simulink model "dvbs2_stream"  (R2024b)
settings: Solver=FixedStepDiscrete  StartTime=0.0  StopTime=18000/Fs  RelTol=1e-3
PreLoadFcn:
  | Rs = 125e3;
  | Fs = 8*Rs;
  | nsamp = 4096;
  | t = (0:nsamp)/Fs;
  | y = randi(2^8-1,1,2048);
  | ly = length(y);
InitFcn:
  | Rs = 125e3;
  | Fs = 8*Rs;
  | nsamp = 4096;
  | t = (0:nsamp)/Fs;
  | y = randi(2^8-1,1,2048);
  | ly = length(y);
libraries: hdlsllib x132, simulink x41, dspsigops x7, commseqgen3 x5, whdlutilities x5, commhdlcrc x2, dsphdlfiltering2 x1, whdlmod x1, sdrzblksprivate x1
(part 1 of 6)
CloseFcn:
  | clear Fs nsamp t y ly
settings Model: Creator=The MathWorks, Inc.  LastModifiedBy=daniel
settings SolverCC: AlgebraicLoopSolver=TrustRegion
settings OptimizationCC: BlockReduction=off  ConditionallyExecuteInputs=off  DefaultParameterBehavior=Inlined
settings DebuggingCC: AlgebraicLoopMsg=error  UnconnectedInputMsg=warning  UnconnectedOutputMsg=warning  UnconnectedLineMsg=warning
settings HardwareCC: ProdBitPerPointer=32  ProdBitPerSizeT=32  ProdBitPerPtrDiffT=32  ProdLargestAtomicFloat=None  ProdIntDivRoundTo=Undefined  ProdEndianess=Unspecified  ProdWordSize=32  ProdHWDeviceType=ASIC/FPGA->ASIC/FPGA  TargetBitPerLong=64  TargetBitPerPointer=64  TargetBitPerSizeT=64  TargetBitPerPtrDiffT=64  TargetLongLongMode=on  TargetIntDivRoundTo=Zero  TargetEndianess=LittleEndian  TargetWordSize=64  TargetHWDeviceType=Custom Processor->MATLAB Host Computer  ProdEqTarget=off
settings ModelReferenceCC: EnableRefExpFcnMdlSchedulingChecks=on
settings RTWCC: GPUComputeCapability=3.5

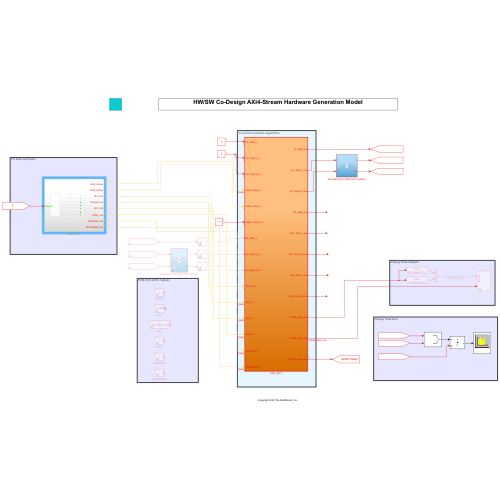
[thumbnail: Simulink's stored preview of the top-level diagram]
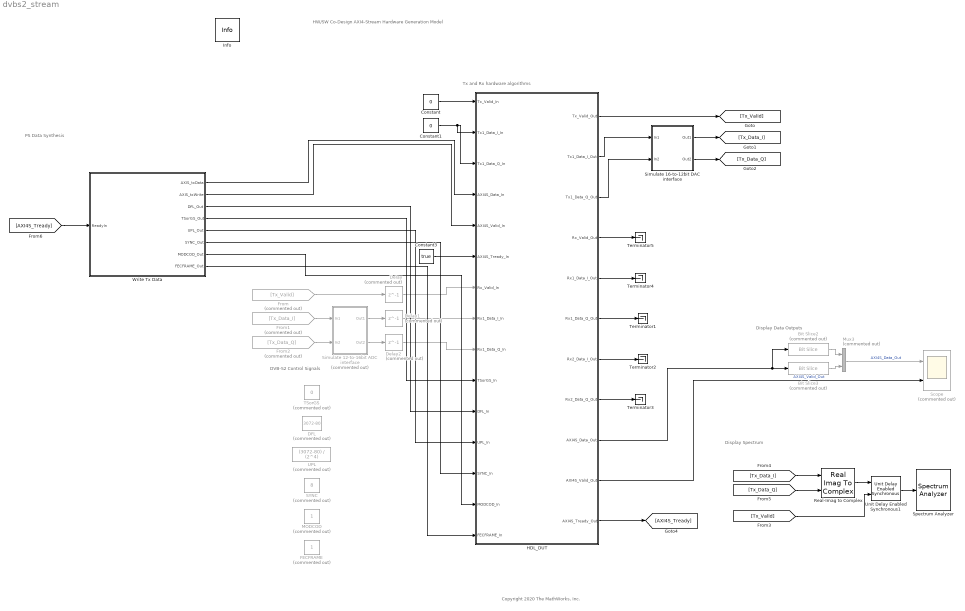
== system dvbs2_stream ==
  note: Tx and Rx hardware algorithms
  note: DVB-S2 Control Signals
  note: Display Data Outputs
  note: PS Data Synthesis
  note: HW/SW Co-Design AXI4-Stream Hardware Generation Model
  note: Copyright 2020 The MathWorks, Inc.
  note: Display Spectrum
  Bit Slice2 : hdlsllib/Logic and Bit Operations/Bit Slice  Commented=on  lidx=31  ridx=16
  Bit Slice3 : hdlsllib/Logic and Bit Operations/Bit Slice  Commented=on  lidx=15  ridx=0
  Constant : Constant  Value=0  OutDataTypeStr=boolean  SampleTime=-1
  Constant1 : Constant  Value=0  OutDataTypeStr=int16  SampleTime=-1
  Constant3 : Constant  Value=true  SampleTime=-1
  DFL : Constant  Commented=on  Value=3072-80  OutDataTypeStr=uint16  SampleTime=-1
  Delay : Delay  Commented=on  DelayLength=1
  Delay1 : Delay  Commented=on  DelayLength=1
  Delay2 : Delay  Commented=on  DelayLength=1
  FECFRAME : Constant  Commented=on  OutDataTypeStr=boolean  SampleTime=-1
  From : From  Commented=on  GotoTag=Tx_Valid
  From1 : From  Commented=on  GotoTag=Tx_Data_I
  From2 : From  Commented=on  GotoTag=Tx_Data_Q
  HDL_DUT : Subsystem  TreatAsAtomicUnit=on
  Info : sdrzblksprivate/Info  SystemSampleTime=-1  VariantActivationTime=update diagram  AllowFlexibleInterface=on  Latency=0  AutoFrameSizeCalculation=off
  MODCOD : Constant  Commented=on  OutDataTypeStr=fixdt(0,5,0)  SampleTime=-1
  Mux3 : Mux  Commented=on  Inputs=2
  Real-Imag to Complex : RealImagToComplex
  SYNC : Constant  Commented=on  Value=8  OutDataTypeStr=uint8  SampleTime=-1
  Scope : Scope  Commented=on  NumInputPorts=2
  Simulate 12-to-16bit ADC interface : Subsystem  Commented=on
  Simulate 16-to-12bit DAC interface : Subsystem
  Spectrum Analyzer : SpectrumAnalyzer  WindowPosition=[97.000000,769.000000,800.000000,500.000000,]  ScopeFrameLocation=window  WindowInvariantSamplesPerUpdate=on  Span=500000  StartFrequency=-250000  StopFrequency=250000  YLimits=[16.077875713171906,86.7369585129505]
  TSorGS : Constant  Commented=on  Value=0  OutDataTypeStr=fixdt(0,2,0)  SampleTime=-1
  Terminator{1..5} (5 alike) : Terminator
  UPL : Constant  Commented=on  Value=(3072-80) / (2^4)  OutDataTypeStr=uint16  SampleTime=-1
  Unit Delay Enabled Synchronous1 : hdlsllib/Discrete/Unit Delay Enabled Synchronous  InitialCondition=0.0  SampleTime=-1
  Write Tx Data : Subsystem
  wires:
  From/1 -> Delay/1
  Bit Slice2/1 -> Mux3/1
  Delay1/1 -> HDL_DUT/8(Rx1_Data_I_In)
  HDL_DUT/1(Tx_Valid_Out) -> [Tx_Valid]
  Constant/1 -> HDL_DUT/1(Tx_Valid_In)
  Delay2/1 -> HDL_DUT/9(Rx1_Data_Q_In)
  Write Tx Data/1(AXIS_txData) -> HDL_DUT/4(AXI4S_Data_In)
  Constant1/1 -> HDL_DUT/2(Tx1_Data_I_In), HDL_DUT/3(Tx1_Data_Q_In)
  Write Tx Data/2(AXIS_txWrite) -> HDL_DUT/5(AXI4S_Valid_In)
  HDL_DUT/10(AXI4S_Valid_Out) -> Scope/2  "AXI4S_Valid_Out"
  Delay/1 -> HDL_DUT/7(Rx_Valid_In)
  HDL_DUT/9(AXI4S_Data_Out) -> Bit Slice2/1, Bit Slice3/1
  HDL_DUT/2(Tx1_Data_I_Out) -> Simulate 16-to-12bit DAC interface/1(In1)
  HDL_DUT/3(Tx1_Data_Q_Out) -> Simulate 16-to-12bit DAC interface/2(In2)
  Simulate 16-to-12bit DAC interface/1(Out1) -> [Tx_Data_I]
  Simulate 16-to-12bit DAC interface/2(Out2) -> [Tx_Data_Q]
  From1/1 -> Simulate 12-to-16bit ADC interface/1(In1)
  From2/1 -> Simulate 12-to-16bit ADC interface/2(In2)
  Simulate 12-to-16bit ADC interface/1(Out1) -> Delay1/1
  Simulate 12-to-16bit ADC interface/2(Out2) -> Delay2/1
  Constant3/1 -> HDL_DUT/6(AXI4S_Tready_In)
  HDL_DUT/11(AXI4S_Tready_Out) -> [AXI4S_Tready]
  Bit Slice3/1 -> Mux3/2
  Mux3/1 -> Scope/1  "AXI4S_Data_Out"
  HDL_DUT/6(Rx1_Data_Q_Out) -> Terminator1/1
  HDL_DUT/7(Rx2_Data_I_Out) -> Terminator2/1
  HDL_DUT/8(Rx2_Data_Q_Out) -> Terminator3/1
  HDL_DUT/5(Rx1_Data_I_Out) -> Terminator4/1
  HDL_DUT/4(Rx_Valid_Out) -> Terminator5/1
  Write Tx Data/4(TSorGS_Out) -> HDL_DUT/10(TSorGS_In)
  Write Tx Data/3(DFL_Out) -> HDL_DUT/11(DFL_In)
  Write Tx Data/5(UPL_Out) -> HDL_DUT/12(UPL_In)
  Write Tx Data/6(SYNC_Out) -> HDL_DUT/13(SYNC_In)
  Write Tx Data/7(MODCOD_Out) -> HDL_DUT/14(MODCOD_In)
  Write Tx Data/8(FECFRAME_Out) -> HDL_DUT/15(FECFRAME_In)
  [Tx_Data_I] -> Real-Imag to Complex/1
  [Tx_Data_Q] -> Real-Imag to Complex/2
  [Tx_Valid] -> Unit Delay Enabled Synchronous1/2
  Real-Imag to Complex/1 -> Unit Delay Enabled Synchronous1/1
  Unit Delay Enabled Synchronous1/1 -> Spectrum Analyzer/1
  [AXI4S_Tready] -> Write Tx Data/1(ReadyIn)

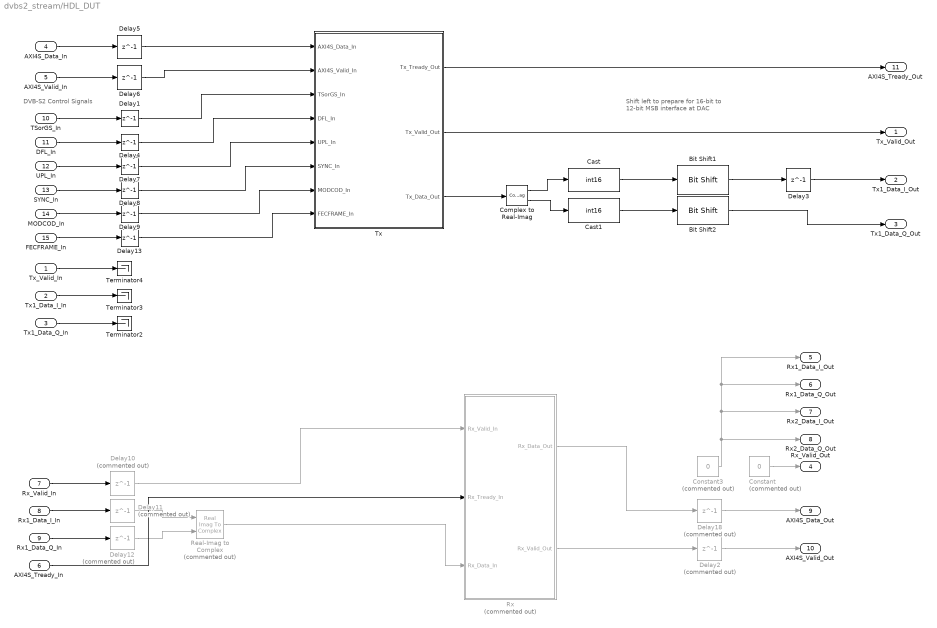
== system dvbs2_stream/HDL_DUT ==
  note: DVB-S2 Control Signals
  note: Shift left to prepare for 16-bit to 12-bit MSB interface at DAC
  Tx_Valid_In : Inport
  Tx1_Data_I_In : Inport  Port=2
  Tx1_Data_Q_In : Inport  Port=3
  AXI4S_Data_In : Inport  Port=4
  AXI4S_Valid_In : Inport  Port=5
  AXI4S_Tready_In : Inport  Port=6
  Rx_Valid_In : Inport  Port=7
  Rx1_Data_I_In : Inport  Port=8
  Rx1_Data_Q_In : Inport  Port=9
  TSorGS_In : Inport  Port=10
  DFL_In : Inport  Port=11
  UPL_In : Inport  Port=12
  SYNC_In : Inport  Port=13
  MODCOD_In : Inport  Port=14
  FECFRAME_In : Inport  Port=15
  Bit Shift1 : hdlsllib/Logic and Bit Operations/Bit Shift  mode=Shift Left Logical  N=4
  Bit Shift2 : hdlsllib/Logic and Bit Operations/Bit Shift  mode=Shift Left Logical  N=4
  Cast : DataTypeConversion  OutDataTypeStr=int16  ConvertRealWorld=Stored Integer (SI)  SaturateOnIntegerOverflow=off  RndMeth=Floor
  Cast1 : DataTypeConversion  OutDataTypeStr=int16  ConvertRealWorld=Stored Integer (SI)  SaturateOnIntegerOverflow=off  RndMeth=Floor
  Complex to Real-Imag : ComplexToRealImag
  Constant : Constant  Commented=on  Value=0  OutDataTypeStr=boolean  SampleTime=-1
  Constant3 : Constant  Commented=on  Value=0  OutDataTypeStr=int16  SampleTime=-1
  Delay{1,3..9,13} (9 alike) : Delay  DelayLength=1
  Delay{2,10..12,18} (5 alike) : Delay  Commented=on  DelayLength=1
  Real-Imag to Complex : RealImagToComplex  Commented=on
  Rx : Subsystem  Commented=on
  Terminator2 : Terminator
  Terminator3 : Terminator
  Terminator4 : Terminator
  Tx : Subsystem
  Tx_Valid_Out : Outport
  Tx1_Data_I_Out : Outport  Port=2
  Tx1_Data_Q_Out : Outport  Port=3
  Rx_Valid_Out : Outport  Port=4
  Rx1_Data_I_Out : Outport  Port=5
  Rx1_Data_Q_Out : Outport  Port=6
  Rx2_Data_I_Out : Outport  Port=7
  Rx2_Data_Q_Out : Outport  Port=8
  AXI4S_Data_Out : Outport  Port=9
  AXI4S_Valid_Out : Outport  Port=10
  AXI4S_Tready_Out : Outport  Port=11
  wires:
  Tx1_Data_I_In/1 -> Terminator3/1
  Tx_Valid_In/1 -> Terminator4/1
  Tx1_Data_Q_In/1 -> Terminator2/1
  AXI4S_Data_In/1 -> Delay5/1
  AXI4S_Valid_In/1 -> Delay6/1
  Delay6/1 -> Tx/2(AXI4S_Valid_In)
  Rx_Valid_In/1 -> Delay10/1
  Rx1_Data_I_In/1 -> Delay11/1
  Rx1_Data_Q_In/1 -> Delay12/1
  Delay5/1 -> Tx/1(AXI4S_Data_In)
  Delay11/1 -> Real-Imag to Complex/1
  Delay12/1 -> Real-Imag to Complex/2
  Delay3/1 -> Tx1_Data_I_Out/1
  Bit Shift2/1 -> Tx1_Data_Q_Out/1
  Constant3/1 -> Rx1_Data_Q_Out/1, Rx1_Data_I_Out/1, Rx2_Data_I_Out/1, Rx2_Data_Q_Out/1
  Delay10/1 -> Rx/1(Rx_Valid_In)
  Real-Imag to Complex/1 -> Rx/3(Rx_Data_In)
  Delay18/1 -> AXI4S_Data_Out/1
  Bit Shift1/1 -> Delay3/1
  Delay2/1 -> AXI4S_Valid_Out/1
  Tx/1(Tx_Tready_Out) -> AXI4S_Tready_Out/1
  AXI4S_Tready_In/1 -> Rx/2(Rx_Tready_In)
  Constant/1 -> Rx_Valid_Out/1
  Tx/2(Tx_Valid_Out) -> Tx_Valid_Out/1
  Rx/1(Rx_Data_Out) -> Delay18/1
  Rx/2(Rx_Valid_Out) -> Delay2/1
  TSorGS_In/1 -> Delay1/1
  DFL_In/1 -> Delay4/1
  UPL_In/1 -> Delay7/1
  SYNC_In/1 -> Delay8/1
  MODCOD_In/1 -> Delay9/1
  FECFRAME_In/1 -> Delay13/1
  Delay1/1 -> Tx/3(TSorGS_In)
  Delay4/1 -> Tx/4(DFL_In)
  Delay7/1 -> Tx/5(UPL_In)
  Delay8/1 -> Tx/6(SYNC_In)
  Delay9/1 -> Tx/7(MODCOD_In)
  Delay13/1 -> Tx/8(FECFRAME_In)
  Tx/3(Tx_Data_Out) -> Complex to Real-Imag/1
  Complex to Real-Imag/1 -> Cast/1
  Complex to Real-Imag/2 -> Cast1/1
  Cast/1 -> Bit Shift1/1
  Cast1/1 -> Bit Shift2/1

== system dvbs2_stream/Simulate 12-to-16bit ADC interface ==
  In1 : Inport
  In2 : Inport  Port=2
  Data Type Conversion : DataTypeConversion  OutDataTypeStr=int16  SaturateOnIntegerOverflow=off  RndMeth=Floor
  Data Type Conversion1 : DataTypeConversion  OutDataTypeStr=int16  SaturateOnIntegerOverflow=off  RndMeth=Floor
  Out1 : Outport
  Out2 : Outport  Port=2
  wires:
  In2/1 -> Data Type Conversion/1
  Data Type Conversion1/1 -> Out1/1
  In1/1 -> Data Type Conversion1/1
  Data Type Conversion/1 -> Out2/1

== system dvbs2_stream/Simulate 16-to-12bit DAC interface ==
  In1 : Inport
  In2 : Inport  Port=2
  Bit Shift1 : hdlsllib/Logic and Bit Operations/Bit Shift  mode=Shift Right Arithmetic  N=4
  Bit Shift2 : hdlsllib/Logic and Bit Operations/Bit Shift  mode=Shift Right Arithmetic  N=4
  Out1 : Outport
  Out2 : Outport  Port=2
  wires:
  In1/1 -> Bit Shift1/1
  In2/1 -> Bit Shift2/1
  Bit Shift1/1 -> Out1/1
  Bit Shift2/1 -> Out2/1

== system dvbs2_stream/Write Tx Data ==
  ReadyIn : Inport
  Constant : Constant
  Generate_Data : MATLAB Function  TreatAsAtomicUnit=on  mask{frm_bits=1, pkt_bits=2, pl_cnt_bits=5, frameEnd_pos=3, frameStart_pos=2, pktEnd_pos=1, pktStart_pos=0, TSorGS_In=0, DFL_In=32*4, UPL_In=32, SYNC_In=0x00, MODCOD_In=0x02, FECFRAME_In=0, nPackets=4, nFrames=4}
      mask prompts: pl_cnt_bits "payload_count_bits"; TSorGS_In "TSorGS"; DFL_In "DFL"; UPL_In "UPL"; SYNC_In "SYNC"; MODCOD_In "MODCOD"; FECFRAME_In "FECFRAME"
  Serializer1D{,1..6} (7 alike) : hdlsllib/HDL Operations/Serializer1D  Ratio=64  IdleCycles=0  validIn=off  startOut=off  validOut=off  inputDataDimensions=-1  inputSampleTime=-1  inputSignalType=auto
  Unit Delay Enabled Synchronous{,1..6} (7 alike) : hdlsllib/Discrete/Unit Delay Enabled Synchronous  InitialCondition=0.0  SampleTime=-1
  AXIS_txData : Outport  SampleTime=1/ Fs
  AXIS_txWrite : Outport  Port=2  SampleTime=1 / Fs
  DFL_Out : Outport  Port=3  SampleTime=1/ Fs
  TSorGS_Out : Outport  Port=4  SampleTime=1 / Fs
  UPL_Out : Outport  Port=5  SampleTime=1/ Fs
  SYNC_Out : Outport  Port=6  SampleTime=1 / Fs
  MODCOD_Out : Outport  Port=7  SampleTime=1/ Fs
  FECFRAME_Out : Outport  Port=8  SampleTime=1 / Fs
  wires:
  ReadyIn/1 -> Unit Delay Enabled Synchronous6/2, Unit Delay Enabled Synchronous5/2, Unit Delay Enabled Synchronous4/2, Unit Delay Enabled Synchronous3/2, Unit Delay Enabled Synchronous2/2, Unit Delay Enabled Synchronous1/2, Unit Delay Enabled Synchronous/2  "ReadySig"
  Generate_Data/7(data_Out) -> Serializer1D6/1  "data"
  Unit Delay Enabled Synchronous/1 -> AXIS_txData/1  "TxData"
  Constant/1 -> AXIS_txWrite/1
  Generate_Data/2(DFL_Out) -> Serializer1D1/1  "DFL"
  Generate_Data/1(TSorGS_Out) -> Serializer1D/1  "TSorGS"
  Generate_Data/3(UPL_Out) -> Serializer1D2/1  "UPL"
  Generate_Data/4(SYNC_Out) -> Serializer1D3/1  "SYNC"
  Generate_Data/5(MODCOD_Out) -> Serializer1D4/1  "MODCOD"
  Generate_Data/6(FECFRAME_Out) -> Serializer1D5/1  "FECFRAME"
  Unit Delay Enabled Synchronous1/1 -> FECFRAME_Out/1  "FECFRAME_en"
  Unit Delay Enabled Synchronous2/1 -> MODCOD_Out/1  "MODCOD_en"
  Unit Delay Enabled Synchronous3/1 -> SYNC_Out/1  "SYNC_en"
  Unit Delay Enabled Synchronous4/1 -> UPL_Out/1  "UPL_en"
  Unit Delay Enabled Synchronous5/1 -> DFL_Out/1  "DFL_en"
  Unit Delay Enabled Synchronous6/1 -> TSorGS_Out/1  "TSGS_en"
  Serializer1D/1 -> Unit Delay Enabled Synchronous6/1
  Serializer1D1/1 -> Unit Delay Enabled Synchronous5/1
  Serializer1D2/1 -> Unit Delay Enabled Synchronous4/1
  Serializer1D3/1 -> Unit Delay Enabled Synchronous3/1
  Serializer1D5/1 -> Unit Delay Enabled Synchronous1/1
  Serializer1D4/1 -> Unit Delay Enabled Synchronous2/1
  Serializer1D6/1 -> Unit Delay Enabled Synchronous/1

== system dvbs2_stream/HDL_DUT/Rx ==
  note: Ignore any Backpressure exerted on DUT
  Rx_Valid_In : Inport
  Rx_Tready_In : Inport  Port=2
  Rx_Data_In : Inport  Port=3
  Terminator1 : Terminator
  Rx_Data_Out : Outport
  Rx_Valid_Out : Outport  Port=2
  wires:
  Rx_Valid_In/1 -> Rx_Valid_Out/1
  Rx_Tready_In/1 -> Terminator1/1
  Rx_Data_In/1 -> Rx_Data_Out/1

== system dvbs2_stream/HDL_DUT/Tx ==
  AXI4S_Data_In : Inport
  AXI4S_Valid_In : Inport  Port=2
  TSorGS_In : Inport  Port=3  OutDataTypeStr=fixdt(0,2,0)
  DFL_In : Inport  Port=4  OutDataTypeStr=uint16
  UPL_In : Inport  Port=5  OutDataTypeStr=uint16
  SYNC_In : Inport  Port=6  OutDataTypeStr=uint8
  MODCOD_In : Inport  Port=7  OutDataTypeStr=fixdt(0,5,0)
  FECFRAME_In : Inport  Port=8  OutDataTypeStr=boolean
  Bit Slice2 : hdlsllib/Logic and Bit Operations/Bit Slice  lidx=0  ridx=0
  Bit Slice3 : hdlsllib/Logic and Bit Operations/Bit Slice  lidx=1  ridx=1
  Bit Slice4 : hdlsllib/Logic and Bit Operations/Bit Slice  lidx=2  ridx=2
  Bit Slice5 : hdlsllib/Logic and Bit Operations/Bit Slice  lidx=3  ridx=3
  Constant2 : Constant  Value=0
  Control : hdlsllib/Logic and Bit Operations/Bit Slice  lidx=3  ridx=0
  DVB-S2 Tx : Subsystem  mask{Rsym=Rs}
      mask prompts: Rsym "Symbol Rate:"
      mask init:
      | config = dvbs2hdlTxParameters();
  Data : hdlsllib/Logic and Bit Operations/Bit Slice  lidx=11  ridx=4
  Data Type Conversion{1..2,4..6} (5 alike) : DataTypeConversion  OutDataTypeStr=boolean  SaturateOnIntegerOverflow=off  RndMeth=Floor
  Delay : Delay  DelayLength=8  InitialCondition=0
  Delay1 : Delay  DelayLength=7  InitialCondition=0
  Delay2 : Delay  DelayLength=5  InitialCondition=0
  MATLAB Function1 : MATLAB Function  TreatAsAtomicUnit=on
  Terminator6 : Terminator
  Terminator7 : Terminator
  Tx_Tready_Out : Outport
  Tx_Valid_Out : Outport  Port=2
  Tx_Data_Out : Outport  Port=3
  wires:
  AXI4S_Data_In/1 -> Data/1, Control/1
  Control/1 -> Delay2/1
  DVB-S2 Tx/1(dataOut) -> Tx_Data_Out/1  "dataOut"
  DVB-S2 Tx/2(validOut) -> Tx_Valid_Out/1  "validOut"
  Bit Slice2/1 -> Data Type Conversion1/1
  Bit Slice3/1 -> Delay/1
  AXI4S_Valid_In/1 -> MATLAB Function1/2(validIn)
  Bit Slice4/1 -> Data Type Conversion4/1
  Bit Slice5/1 -> Delay1/1
  DFL_In/1 -> DVB-S2 Tx/8(DFL)  "DFL"
  UPL_In/1 -> DVB-S2 Tx/9(UPL)  "UPL"
  SYNC_In/1 -> DVB-S2 Tx/10(SYNC)  "SYNC"
  MODCOD_In/1 -> DVB-S2 Tx/11(pMODCOD)  "pMODCOD"
  TSorGS_In/1 -> DVB-S2 Tx/7(TSorGS)  "TSorGS"
  FECFRAME_In/1 -> DVB-S2 Tx/12(pFECFrame)  "pFECFRAME"
  Delay/1 -> Data Type Conversion2/1
  Delay1/1 -> Data Type Conversion5/1
  DVB-S2 Tx/3(flag) -> Terminator6/1  "flag"
  DVB-S2 Tx/4(nextFrame) -> Terminator7/1  "nextFrame"
  MATLAB Function1/3(readyOut) -> Tx_Tready_Out/1
  Data Type Conversion1/1 -> DVB-S2 Tx/2(pktStartIn)  "pktStartIn"
  Data Type Conversion2/1 -> DVB-S2 Tx/3(pktEndIn)  "pktEndIn"
  MATLAB Function1/2(pktValidOut) -> DVB-S2 Tx/4(pktValidIn)  "pktValidIn"
  Data Type Conversion4/1 -> DVB-S2 Tx/5(frameStartIn)  "frameStartIn"
  Data Type Conversion5/1 -> DVB-S2 Tx/6(frameEndIn)  "frameEndIn"
  Data/1 -> MATLAB Function1/1(byteIn)  "byteIn"
  MATLAB Function1/1(pktBitOut) -> Data Type Conversion6/1
  Data Type Conversion6/1 -> DVB-S2 Tx/1(pktBitsIn)  "pktBitsIn"
  Constant2/1 -> MATLAB Function1/3(LSBfirst)
  Delay2/1 -> Bit Slice5/1, Bit Slice4/1, Bit Slice3/1, Bit Slice2/1

== system dvbs2_stream/HDL_DUT/Tx/DVB-S2 Tx ==
  pktBitsIn : Inport  SampleTime=1/(Rsym*8)
  pktStartIn : Inport  Port=2  SampleTime=1/(Rsym*8)
  pktEndIn : Inport  Port=3  SampleTime=1/(Rsym*8)
  pktValidIn : Inport  Port=4  SampleTime=1/(Rsym*8)
  frameStartIn : Inport  Port=5  SampleTime=1/(Rsym*8)
  frameEndIn : Inport  Port=6  SampleTime=1/(Rsym*8)
  TSorGS : Inport  Port=7  SampleTime=1/(Rsym*8)
  DFL : Inport  Port=8  SampleTime=1/(Rsym*8)
  UPL : Inport  Port=9  SampleTime=1/(Rsym*8)
  SYNC : Inport  Port=10  SampleTime=1/(Rsym*8)
  pMODCOD : Inport  Port=11  SampleTime=1/(Rsym*8)
  pFECFrame : Inport  Port=12  SampleTime=1/(Rsym*8)
  BB Frame Generator : Subsystem
  Bit Concat : hdlsllib/Logic and Bit Operations/Bit Concat  numInputs=2
  Delay : Delay  DelayLength=1
  FEC Encoder : Subsystem
  Interleaver : Subsystem
  Logical Operator : Logic  Operator=NOT  AllPortsSameDT=off  OutDataTypeStr=boolean
  Logical Operator1 : Logic  AllPortsSameDT=off  OutDataTypeStr=boolean
  MODCOD Source Coder : Subsystem
  No HDL : Subsystem
  PL Frame Generator : Subsystem
  RRC Transmit Filter : Subsystem
  Symbol Modulator : Subsystem
  Unit Delay Enabled Resettable Synchronous : hdlsllib/Discrete/Unit Delay Enabled Resettable Synchronous  InitialCondition=0.0  SampleTime=-1
  dataOut : Outport
  validOut : Outport  Port=2
  flag : Outport  Port=3
  nextFrame : Outport  Port=4
  wires:
  BB Frame Generator/4(validOut) -> MODCOD Source Coder/4(validIn)
  Delay/1 -> Logical Operator/1
  Logical Operator/1 -> Logical Operator1/2
  Logical Operator1/1 -> Unit Delay Enabled Resettable Synchronous/2, Unit Delay Enabled Resettable Synchronous/1
  PL Frame Generator/4(PLHeaderEnd) -> Bit Concat/2, No HDL/2(enb)
  PL Frame Generator/3(dummyHeaderEnd) -> Bit Concat/1, No HDL/1(Enable)
  Interleaver/8(MODCOD) -> Symbol Modulator/8(MODCOD)
  Interleaver/7(modIdx) -> Symbol Modulator/7(modIdx)
  Interleaver/6(codIdx) -> Symbol Modulator/6(codIdx)
  Interleaver/5(FECFrame) -> Symbol Modulator/5(FECFrame)
  Interleaver/4(validOut) -> Symbol Modulator/4(validIn)
  Interleaver/3(endOut) -> Symbol Modulator/3(endIn)
  Interleaver/2(startOut) -> Symbol Modulator/2(startIn)
  Interleaver/1(dataOut) -> Symbol Modulator/1(dataIn)
  FEC Encoder/7(MODCOD) -> Interleaver/7(MODCODIn)
  FEC Encoder/5(codOut) -> Interleaver/5(codIdxIn)
  FEC Encoder/2(validOut) -> Interleaver/2(validIn)
  FEC Encoder/1(dataOut) -> Interleaver/1(dataIn)
  PL Frame Generator/2(validOut) -> RRC Transmit Filter/2(validIn)
  PL Frame Generator/1(dataOut) -> RRC Transmit Filter/1(dataIn)
  Symbol Modulator/8(MODCODOut) -> PL Frame Generator/8(modcod)
  Symbol Modulator/7(FECFrameOut) -> PL Frame Generator/7(fecframeIn)
  Symbol Modulator/6(codIdxOut) -> PL Frame Generator/6(codIdxIn)
  Symbol Modulator/5(modIdxOut) -> PL Frame Generator/5(modIdxIn)
  Symbol Modulator/4(validOut) -> PL Frame Generator/4(validIn)
  Symbol Modulator/3(endOut) -> PL Frame Generator/3(endIn)
  Symbol Modulator/2(startOut) -> PL Frame Generator/2(startIn)
  Symbol Modulator/1(dataOut) -> PL Frame Generator/1(dataIn)
  RRC Transmit Filter/2(validOut) -> validOut/1
  RRC Transmit Filter/1(dataOut) -> dataOut/1
  pFECFrame/1 -> BB Frame Generator/12(pFECFrame)  "pFECFRAME"
  Interleaver/9(ready) -> Delay/1, Logical Operator1/1
  frameEndIn/1 -> BB Frame Generator/6(frameEndIn)  "frameEndIn"
  TSorGS/1 -> BB Frame Generator/7(TSorGS)  "TSorGS"
  pktBitsIn/1 -> BB Frame Generator/1(pktBitsIn)  "pktBitsIn"
  pktEndIn/1 -> BB Frame Generator/3(pktEndIn)  "pktEndIn"
  DFL/1 -> BB Frame Generator/8(DFL)  "DFL"
  FEC Encoder/3(startOut) -> Interleaver/3(paramValid)
  MODCOD Source Coder/4(validOut) -> FEC Encoder/4(validIn)
  pktValidIn/1 -> BB Frame Generator/4(pktValidIn)  "pktValidIn"
  MODCOD Source Coder/1(dataOut) -> FEC Encoder/1(dataIn)
  MODCOD Source Coder/3(endOut) -> FEC Encoder/3(endIn)
  MODCOD Source Coder/8(MODCOD) -> FEC Encoder/8(MODCODIn)
  BB Frame Generator/6(FECFrame) -> MODCOD Source Coder/6(FECFrameIn)
  BB Frame Generator/1(dataOut) -> MODCOD Source Coder/1(dataIn)
  pMODCOD/1 -> BB Frame Generator/11(pMODCOD)  "pMODCOD"
  MODCOD Source Coder/2(startOut) -> FEC Encoder/2(startIn)
  MODCOD Source Coder/6(codeRateIdx) -> FEC Encoder/6(codeRateIdxIn)
  SYNC/1 -> BB Frame Generator/10(SYNC)  "SYNC"
  UPL/1 -> BB Frame Generator/9(UPL)  "UPL"
  BB Frame Generator/2(startOut) -> MODCOD Source Coder/2(startIn)
  pktStartIn/1 -> BB Frame Generator/2(pktStartIn)  "pktStartIn"
  BB Frame Generator/5(MODCOD) -> MODCOD Source Coder/5(MODCODIn)
  MODCOD Source Coder/5(modIdx) -> FEC Encoder/5(modIdxIn)
  MODCOD Source Coder/7(FECFrame) -> FEC Encoder/7(FECFrameIn)
  frameStartIn/1 -> Unit Delay Enabled Resettable Synchronous/3, BB Frame Generator/5(frameStartIn)  "frameStartIn"
  FEC Encoder/4(modOut) -> Interleaver/4(modIdxIn)
  BB Frame Generator/3(endOut) -> MODCOD Source Coder/3(endIn)
  FEC Encoder/6(fecOut) -> Interleaver/6(fecframeIn)
  Unit Delay Enabled Resettable Synchronous/1 -> nextFrame/1
  Bit Concat/1 -> flag/1

== system dvbs2_stream/HDL_DUT/Tx/DVB-S2 Tx/BB Frame Generator ==
  pktBitsIn : Inport
  pktStartIn : Inport  Port=2
  pktEndIn : Inport  Port=3
  pktValidIn : Inport  Port=4
  frameStartIn : Inport  Port=5
  frameEndIn : Inport  Port=6
  TSorGS : Inport  Port=7
  DFL : Inport  Port=8
  UPL : Inport  Port=9
  SYNC : Inport  Port=10
  pMODCOD : Inport  Port=11
  pFECFrame : Inport  Port=12
  BB Header and Data CRC Generator : Subsystem
  BB Scrambler : Subsystem
  Data Store FIFO : Subsystem
  Delay{,1..2,5} (4 alike) : Delay  DelayLength=1
  Multiplexer : Subsystem
  Unit Delay Enabled Synchronous{,1..5} (6 alike) : hdlsllib/Discrete/Unit Delay Enabled Synchronous  InitialCondition=0.0  SampleTime=-1
  dataOut : Outport
  startOut : Outport  Port=2
  endOut : Outport  Port=3
  validOut : Outport  Port=4
  MODCOD : Outport  Port=5
  FECFrame : Outport  Port=6
  wires:
  BB Scrambler/6(FECFrameOut) -> FECFrame/1
  Multiplexer/6(FECFrameOut) -> BB Scrambler/6(FECFrame)
  Data Store FIFO/8(FECFrameOut) -> Multiplexer/8(FECFrame)
  BB Header and Data CRC Generator/9(FECFrameOut) -> Data Store FIFO/9(FECFrame)
  Unit Delay Enabled Synchronous5/1 -> BB Header and Data CRC Generator/12(FECFrame)
  pFECFrame/1 -> Unit Delay Enabled Synchronous5/1
  BB Scrambler/5(MODCODOut) -> MODCOD/1
  Multiplexer/5(MODCODOut) -> BB Scrambler/5(MODCOD)
  Data Store FIFO/7(MODCODOut) -> Multiplexer/7(MODCOD)
  BB Header and Data CRC Generator/8(MODCODOut) -> Data Store FIFO/8(MODCOD)
  pMODCOD/1 -> Unit Delay Enabled Synchronous4/1
  Unit Delay Enabled Synchronous4/1 -> BB Header and Data CRC Generator/11(MODCOD)
  BB Header and Data CRC Generator/7(validOut) -> Data Store FIFO/7(validOut)
  BB Header and Data CRC Generator/6(endOut) -> Data Store FIFO/6(endOut)
  BB Header and Data CRC Generator/5(startOut) -> Data Store FIFO/5(startOut)
  BB Header and Data CRC Generator/4(bitsOut) -> Data Store FIFO/4(bitsOut)
  Data Store FIFO/6(headerValid) -> Multiplexer/6(headerValid)
  Data Store FIFO/5(headerStart) -> Multiplexer/5(headerStart)
  Data Store FIFO/4(headerBits) -> Multiplexer/4(headerBits)
  Data Store FIFO/3(dataEnd) -> Multiplexer/3(dataEnd)
  Data Store FIFO/2(dataValid) -> Multiplexer/2(dataValid)
  Data Store FIFO/1(dataBits) -> Multiplexer/1(dataBits)
  BB Header and Data CRC Generator/3(DFLOut) -> Data Store FIFO/3(DFLOut)
  BB Header and Data CRC Generator/2(pktValid) -> Data Store FIFO/2(pktValid)
  BB Header and Data CRC Generator/1(pktBits) -> Data Store FIFO/1(pktBits)
  Unit Delay Enabled Synchronous3/1 -> BB Header and Data CRC Generator/10(SYNC)
  Unit Delay Enabled Synchronous2/1 -> BB Header and Data CRC Generator/9(UPL)
  Unit Delay Enabled Synchronous/1 -> BB Header and Data CRC Generator/8(DFL)
  Unit Delay Enabled Synchronous1/1 -> BB Header and Data CRC Generator/7(TSorGS)
  Delay2/1 -> BB Header and Data CRC Generator/6(frameStart)
  Delay/1 -> BB Header and Data CRC Generator/5(frameEnd)
  Delay1/1 -> BB Header and Data CRC Generator/4(validIn)
  Delay5/1 -> BB Header and Data CRC Generator/1(dataIn)
  BB Scrambler/4(validOut) -> validOut/1
  BB Scrambler/3(endOut) -> endOut/1
  BB Scrambler/2(startOut) -> startOut/1
  BB Scrambler/1(bitsOut) -> dataOut/1
  Multiplexer/1(dataOut) -> BB Scrambler/1(bitsIn)
  Multiplexer/3(endOut) -> BB Scrambler/3(endIn)
  Multiplexer/2(startOut) -> BB Scrambler/2(startIn)
  Multiplexer/4(validOut) -> BB Scrambler/4(validIn)
  frameStartIn/1 -> Delay2/1, Unit Delay Enabled Synchronous1/2, Unit Delay Enabled Synchronous/2, Unit Delay Enabled Synchronous2/2, Unit Delay Enabled Synchronous3/2, Unit Delay Enabled Synchronous4/2, Unit Delay Enabled Synchronous5/2
  pktBitsIn/1 -> Delay5/1
  pktValidIn/1 -> Delay1/1
  frameEndIn/1 -> Delay/1
  DFL/1 -> Unit Delay Enabled Synchronous/1
  UPL/1 -> Unit Delay Enabled Synchronous2/1
  SYNC/1 -> Unit Delay Enabled Synchronous3/1
  pktStartIn/1 -> BB Header and Data CRC Generator/2(startIn)
  pktEndIn/1 -> BB Header and Data CRC Generator/3(endIn)
  TSorGS/1 -> Unit Delay Enabled Synchronous1/1

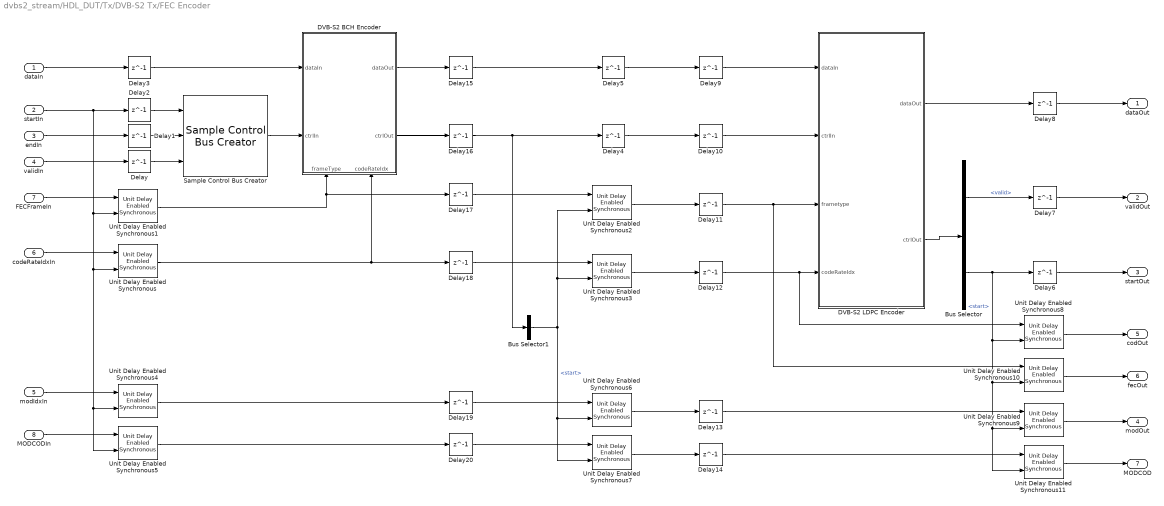
== system dvbs2_stream/HDL_DUT/Tx/DVB-S2 Tx/FEC Encoder ==
  dataIn : Inport
  startIn : Inport  Port=2
  endIn : Inport  Port=3
  validIn : Inport  Port=4
  modIdxIn : Inport  Port=5
  codeRateIdxIn : Inport  Port=6
  FECFrameIn : Inport  Port=7
  MODCODIn : Inport  Port=8
  Bus Selector : BusSelector  OutputSignals=valid,start
  Bus Selector1 : BusSelector  OutputSignals=start
  DVB-S2 BCH Encoder : Subsystem
      settings: PortSchema="{\"entries\":[{\"content\":{\"sides\":[{\"content\":{\"connectorIds\":[\"In1\",\"In2\"]},\"type\":\"ConnectorPlacement.EquallySpacedRectSide\",\"uuid\":\"13af3286-4637-4d72-a307-8c85e9ac2c6a\"},{\"content\":{\"connectorIds\":[\"Out1\",\"Out2\"],\"side\":\"RIGHT\"},\"type\":\"ConnectorPlacement.EquallySpacedRectSide\",\"uuid\":\"54f73aa5-b2da-4ba3-a1a2-5182494cfccf\"},{\"content\":{\"connectorIds\":[],\"side\":\"TOP\"},\"type\":\"ConnectorPlacement.EquallySpacedRectSide\",\"uuid\":\"2ea82380-bfbe-4164-83be-b799e77a8d24\"},{\"content\":{\"connectorIds\":[\"In3\",\"In4\"],\"side\":\"BOTTOM\"},\"type\":\"ConnectorPlacement.EquallySpacedRectSide\",\"uuid\":\"b02c2a1c-1695-4c1d-92ad-7323b1632720\"}]},\"type\":\"ConnectorPlacement.EquallySpacedConnector\",\"uuid\":\"56402870-0df7-4074-88cd-682c42d8a6b3\"}],\"packageUris\":[\"http://schema.mathworks.com/mf0/Connector/R2020b\"],\"version\":\"1.0\"}"
  DVB-S2 LDPC Encoder : Subsystem
      mask init:
      | config = dvbs2hdlTxParameters();
      | columnSum = config.LDPCcolumnSum;  %#ok<NASGU> 
      | ramLUT    = config.LDPCramLUT;     %#ok<NASGU> 
      | shiftLUT  = config.LDPCshiftLUT;   %#ok<NASGU>
  Delay{,1..20} (21 alike) : Delay  DelayLength=1
  Sample Control Bus Creator : whdlutilities/Sample Control Bus Creator
  Unit Delay Enabled Synchronous{,1..11} (12 alike) : hdlsllib/Discrete/Unit Delay Enabled Synchronous  InitialCondition=0.0  SampleTime=-1
  dataOut : Outport
  validOut : Outport  Port=2
  startOut : Outport  Port=3
  modOut : Outport  Port=4
  codOut : Outport  Port=5
  fecOut : Outport  Port=6
  MODCOD : Outport  Port=7
  wires:
  Delay20/1 -> Unit Delay Enabled Synchronous7/1
  Delay19/1 -> Unit Delay Enabled Synchronous6/1
  Delay18/1 -> Unit Delay Enabled Synchronous3/1
  Delay17/1 -> Unit Delay Enabled Synchronous2/1
  Delay16/1 -> Delay4/1, Bus Selector1/1
  Delay15/1 -> Delay5/1
  Delay14/1 -> Unit Delay Enabled Synchronous11/1
  Delay13/1 -> Unit Delay Enabled Synchronous9/1
  Delay12/1 -> DVB-S2 LDPC Encoder/4(codeRateIdx), Unit Delay Enabled Synchronous8/1
  Delay11/1 -> DVB-S2 LDPC Encoder/3(frametype), Unit Delay Enabled Synchronous10/1
  Delay10/1 -> DVB-S2 LDPC Encoder/2(ctrlIn)
  Delay9/1 -> DVB-S2 LDPC Encoder/1(dataIn)
  validIn/1 -> Delay/1
  endIn/1 -> Delay1/1
  startIn/1 -> Delay2/1, Unit Delay Enabled Synchronous1/2, Unit Delay Enabled Synchronous/2, Unit Delay Enabled Synchronous4/2, Unit Delay Enabled Synchronous5/2
  Delay3/1 -> DVB-S2 BCH Encoder/1(dataIn)
  Unit Delay Enabled Synchronous1/1 -> Delay17/1, DVB-S2 BCH Encoder/3(frameType)
  Unit Delay Enabled Synchronous/1 -> DVB-S2 BCH Encoder/4(codeRateIdx), Delay18/1
  Sample Control Bus Creator/1 -> DVB-S2 BCH Encoder/2(ctrlIn)
  DVB-S2 BCH Encoder/2(ctrlOut) -> Delay16/1
  DVB-S2 BCH Encoder/1(dataOut) -> Delay15/1
  Unit Delay Enabled Synchronous3/1 -> Delay12/1
  Delay8/1 -> dataOut/1
  Delay7/1 -> validOut/1
  Delay6/1 -> startOut/1
  Delay5/1 -> Delay9/1
  Delay4/1 -> Delay10/1
  Delay2/1 -> Sample Control Bus Creator/1
  Delay1/1 -> Sample Control Bus Creator/2
  Delay/1 -> Sample Control Bus Creator/3
  Unit Delay Enabled Synchronous7/1 -> Delay14/1
  Unit Delay Enabled Synchronous6/1 -> Delay13/1
  Unit Delay Enabled Synchronous11/1 -> MODCOD/1
  Unit Delay Enabled Synchronous10/1 -> fecOut/1
  Unit Delay Enabled Synchronous9/1 -> modOut/1
  Unit Delay Enabled Synchronous8/1 -> codOut/1
  Unit Delay Enabled Synchronous5/1 -> Delay20/1
  Unit Delay Enabled Synchronous4/1 -> Delay19/1
  MODCODIn/1 -> Unit Delay Enabled Synchronous5/1
  Unit Delay Enabled Synchronous2/1 -> Delay11/1
  Bus Selector1/1 -> Unit Delay Enabled Synchronous6/2, Unit Delay Enabled Synchronous7/2, Unit Delay Enabled Synchronous3/2, Unit Delay Enabled Synchronous2/2  "<start>"
  dataIn/1 -> Delay3/1
  codeRateIdxIn/1 -> Unit Delay Enabled Synchronous/1
  FECFrameIn/1 -> Unit Delay Enabled Synchronous1/1
  modIdxIn/1 -> Unit Delay Enabled Synchronous4/1
  Bus Selector/2 -> Delay6/1, Unit Delay Enabled Synchronous8/2, Unit Delay Enabled Synchronous10/2, Unit Delay Enabled Synchronous9/2, Unit Delay Enabled Synchronous11/2  "<start>"
  Bus Selector/1 -> Delay7/1  "<valid>"
  DVB-S2 LDPC Encoder/2(ctrlOut) -> Bus Selector/1
  DVB-S2 LDPC Encoder/1(dataOut) -> Delay8/1

== system dvbs2_stream/HDL_DUT/Tx/DVB-S2 Tx/Interleaver ==
  dataIn : Inport
  validIn : Inport  Port=2
  paramValid : Inport  Port=3
  modIdxIn : Inport  Port=4
  codIdxIn : Inport  Port=5
  fecframeIn : Inport  Port=6
  MODCODIn : Inport  Port=7
  DVB-S2 HDL Interleaver : Subsystem  mask{mode=Interleaver 8x, Tsamp=1/(Rsym*8)}
      mask prompts: mode "Mode :"; Tsamp "Sample Time"
      mask init:
      | switch mode
      |     case 1
      |         isInterleave = true;
      |     case 2
      |         isInterleave = false;
      |     otherwise
      |         error(['Invalid mode of ' mode]);
      | end
      | clear mode;
      | 
      | ConfigRx.RAMCapacity = 64800*2;
      | ConfigRx.ShortFrameLen = 16200;
      | ConfigRx.NormalFrameLen = 64800;
      mask TypeOptions mode: Interleaver 8x | Deinterleaver
      mask Display: disp(['DVB-S2' newline 'HDL ' newline get_param(gcb,'mode')]);
  Delay{1,3..5,17..20} (8 alike) : Delay  DelayLength=8
  Delay{2,6..13} (9 alike) : Delay  DelayLength=1
  Unit Delay Enabled Synchronous : hdlsllib/Discrete/Unit Delay Enabled Synchronous  InitialCondition=0.0  SampleTime=-1
  dataOut : Outport
  startOut : Outport  Port=2
  endOut : Outport  Port=3
  validOut : Outport  Port=4
  FECFrame : Outport  Port=5
  codIdx : Outport  Port=6
  modIdx : Outport  Port=7
  MODCOD : Outport  Port=8
  ready : Outport  Port=9
  wires:
  Delay1/1 -> endOut/1
  fecframeIn/1 -> DVB-S2 HDL Interleaver/6(fecframeIn)
  modIdxIn/1 -> DVB-S2 HDL Interleaver/4(modIdxIn)
  codIdxIn/1 -> DVB-S2 HDL Interleaver/5(codIdxIn)
  Delay4/1 -> validOut/1
  DVB-S2 HDL Interleaver/8(ready) -> ready/1
  MODCODIn/1 -> Unit Delay Enabled Synchronous/1
  Delay17/1 -> FECFrame/1
  Delay5/1 -> startOut/1
  Delay10/1 -> DVB-S2 HDL Interleaver/2(validIn)
  Delay19/1 -> dataOut/1
  Delay12/1 -> Delay18/1
  dataIn/1 -> Delay9/1
  Delay20/1 -> modIdx/1
  DVB-S2 HDL Interleaver/1(rd_dout) -> Delay2/1
  Delay11/1 -> Delay17/1
  validIn/1 -> Delay10/1
  Delay9/1 -> DVB-S2 HDL Interleaver/1(dataIn)
  Delay8/1 -> Delay4/1
  Delay2/1 -> Delay19/1
  Unit Delay Enabled Synchronous/1 -> Delay3/1
  DVB-S2 HDL Interleaver/2(rd_startOut) -> Delay6/1, Unit Delay Enabled Synchronous/2
  DVB-S2 HDL Interleaver/6(codIdx) -> Delay12/1
  DVB-S2 HDL Interleaver/3(rd_endOut) -> Delay7/1
  Delay3/1 -> MODCOD/1
  Delay6/1 -> Delay5/1
  Delay18/1 -> codIdx/1
  DVB-S2 HDL Interleaver/7(modIdx) -> Delay13/1
  Delay7/1 -> Delay1/1
  paramValid/1 -> DVB-S2 HDL Interleaver/3(paramValid)
  DVB-S2 HDL Interleaver/4(rd_validOut) -> Delay8/1
  DVB-S2 HDL Interleaver/5(fecframe) -> Delay11/1
  Delay13/1 -> Delay20/1

== system dvbs2_stream/HDL_DUT/Tx/DVB-S2 Tx/MODCOD Source Coder ==
  dataIn : Inport
  startIn : Inport  Port=2
  endIn : Inport  Port=3
  validIn : Inport  Port=4
  MODCODIn : Inport  Port=5
  FECFrameIn : Inport  Port=6
  Data Type Conversion : DataTypeConversion  OutDataTypeStr=fixdt(0,4,0)  SaturateOnIntegerOverflow=off  RndMeth=Floor
  Data Type Conversion1 : DataTypeConversion  OutDataTypeStr=boolean  SaturateOnIntegerOverflow=off  RndMeth=Floor
  Data Type Conversion2 : DataTypeConversion  OutDataTypeStr=fixdt(0,2,0)  SaturateOnIntegerOverflow=off  RndMeth=Floor
  Data Type Conversion3 : DataTypeConversion  OutDataTypeStr=fixdt(0,5,0)  SaturateOnIntegerOverflow=off  RndMeth=Floor
  Delay{7..8,14..16} (5 alike) : Delay  DelayLength=1
  Unit Delay Enabled Synchronous : hdlsllib/Discrete/Unit Delay Enabled Synchronous  InitialCondition=0.0  SampleTime=-1
  convertMODCOD : MATLAB Function  TreatAsAtomicUnit=on
  dataOut : Outport
  startOut : Outport  Port=2
  endOut : Outport  Port=3
  validOut : Outport  Port=4
  modIdx : Outport  Port=5
  codeRateIdx : Outport  Port=6
  FECFrame : Outport  Port=7
  MODCOD : Outport  Port=8
  wires:
  Data Type Conversion2/1 -> modIdx/1
  Data Type Conversion1/1 -> FECFrame/1
  Data Type Conversion/1 -> codeRateIdx/1
  Delay7/1 -> dataOut/1
  Delay8/1 -> startOut/1
  endIn/1 -> Delay14/1
  Data Type Conversion3/1 -> MODCOD/1
  validIn/1 -> Delay15/1
  dataIn/1 -> Delay7/1
  Delay14/1 -> endOut/1
  FECFrameIn/1 -> Delay16/1
  convertMODCOD/1(modIdx) -> Data Type Conversion2/1
  MODCODIn/1 -> Unit Delay Enabled Synchronous/1
  Delay15/1 -> validOut/1
  Unit Delay Enabled Synchronous/1 -> convertMODCOD/1(modcod), Data Type Conversion3/1
  convertMODCOD/2(codIdx) -> Data Type Conversion/1
  startIn/1 -> Delay8/1, Unit Delay Enabled Synchronous/2
  Delay16/1 -> Data Type Conversion1/1

== system dvbs2_stream/HDL_DUT/Tx/DVB-S2 Tx/No HDL ==
  Enable : Inport
  enb : Inport  Port=2
  HDL Counter : hdlsllib/Sources/HDL Counter  CountType=Free running  CountInit=0  CountStep=1  CountMax=25  CountFromType=Initial value  CountFrom=0  CountResetPort=off  CountLoadPort=off  CountEnbPort=on  CountDirPort=off  CountHitOutputPort=off  CountDataType=Unsigned  CountWordLen=32  CountFracLen=0  CountSampTime=1
  Subsystem : Subsystem
  wires:
  Enable/1 -> Subsystem/Enable
  enb/1 -> HDL Counter/1
  HDL Counter/1 -> Subsystem/1(In1)

== system dvbs2_stream/HDL_DUT/Tx/DVB-S2 Tx/PL Frame Generator ==
  dataIn : Inport
  startIn : Inport  Port=2
  endIn : Inport  Port=3
  validIn : Inport  Port=4
  modIdxIn : Inport  Port=5
  codIdxIn : Inport  Port=6
  fecframeIn : Inport  Port=7
  modcod : Inport  Port=8
  16x : MATLAB Function  TreatAsAtomicUnit=on
  Constant2 : Constant  Value=true  SampleTime=2/(Rsym)
  Delay : Delay  DelayLength=1
  Delay{1,3,7..11} (7 alike) : Delay  DelayLength=37
  Delay2 : Delay  DelayLength=1
  Downsample : DownSample  N=16  RateOptions=Allow multirate processing
  Downsample{1..2,5..6} (4 alike) : DownSample  N=8  RateOptions=Allow multirate processing
  Downsample3 : DownSample  N=16  RateOptions=Allow multirate processing
  Downsample4 : DownSample  N=16  RateOptions=Allow multirate processing
  Frame Length : Subsystem
  Multiplexer : Subsystem
  PL Data Scrambler : Subsystem
  PL Header Generator : Subsystem
  RAM FIFO : Subsystem
  Subsystem : Subsystem
  Terminator : Terminator
  dataOut : Outport
  validOut : Outport  Port=2
  dummyHeaderEnd : Outport  Port=3
  PLHeaderEnd : Outport  Port=4
  wires:
  16x/1(validOut) -> Downsample/1
  Constant2/1 -> PL Header Generator/2(pilotActive)
  Downsample/1 -> PL Header Generator/1(trigger)
  modcod/1 -> Downsample4/1
  startIn/1 -> Delay1/1, 16x/1(trigger)
  Delay2/1 -> RAM FIFO/2(validIn)
  modIdxIn/1 -> Delay9/1
  PL Header Generator/2(validOut) -> Delay2/1
  PL Header Generator/1(dataOut) -> Delay/1
  codIdxIn/1 -> Delay10/1
  fecframeIn/1 -> Delay11/1, Downsample3/1
  validIn/1 -> Delay8/1
  dataIn/1 -> Delay7/1
  Downsample3/1 -> PL Header Generator/4(fecframe)
  Downsample4/1 -> PL Header Generator/3(modcod)
  Frame Length/1(xFECFrameLength) -> Downsample5/1
  RAM FIFO/10(slotsValid) -> Multiplexer/10(slotsValid)
  RAM FIFO/7(pilotValid) -> Multiplexer/7(pilotValid)
  RAM FIFO/4(plheaderValid) -> Multiplexer/4(plheaderValid)
  Delay/1 -> RAM FIFO/1(dataIn)
  Downsample1/1 -> RAM FIFO/3(dataIn1)
  Downsample2/1 -> RAM FIFO/5(validIn1)
  Downsample5/1 -> RAM FIFO/6(frameLength)
  Downsample6/1 -> RAM FIFO/4(startIn1)
  RAM FIFO/1(plheaderData) -> Multiplexer/1(plheaderData)
  RAM FIFO/2(plheaderStart) -> Multiplexer/2(plheaderStart)
  RAM FIFO/5(pilotData) -> Multiplexer/5(pilotdata)
  RAM FIFO/6(pilotEnd) -> Multiplexer/6(pilotEnd)
  RAM FIFO/8(slotsData) -> Multiplexer/8(slotsData)
  RAM FIFO/9(data16SlotsEnd) -> Multiplexer/9(data16SlotsEnd)
  RAM FIFO/3(plheaderEnd) -> Multiplexer/3(plheaderEnd), PLHeaderEnd/1
  Delay11/1 -> Frame Length/1(fecframe)
  Delay9/1 -> Frame Length/2(modIdx)
  Delay10/1 -> Terminator/1
  Delay7/1 -> Subsystem/1(data)
  Delay1/1 -> Subsystem/2(start)
  Delay8/1 -> Subsystem/4(validIn)
  Subsystem/1(dataOut) -> Downsample1/1
  Subsystem/2(startOut) -> Downsample6/1
  Subsystem/3(validOut) -> Downsample2/1
  endIn/1 -> Delay3/1
  Delay3/1 -> Subsystem/3(endIn)
  RAM FIFO/11(dummyData) -> Multiplexer/11(dummyData)
  RAM FIFO/12(dummyValid) -> Multiplexer/12(dummyValid)
  RAM FIFO/13(dummyHeaderSrt) -> Multiplexer/13(dummyHeaderSrt)
  RAM FIFO/14(dummyHeaderEnd) -> Multiplexer/14(dummyHeaderEnd), dummyHeaderEnd/1
  PL Data Scrambler/2(validOut) -> validOut/1
  Multiplexer/3(endOfPlheader) -> PL Data Scrambler/3(endOfPlheader)
  Multiplexer/2(startOfPlheader) -> PL Data Scrambler/2(startOfPlheader)
  Multiplexer/4(validOut) -> PL Data Scrambler/4(validIn)
  PL Data Scrambler/1(dataOut) -> dataOut/1
  Multiplexer/1(dataOut) -> PL Data Scrambler/1(dataIn)

== system dvbs2_stream/HDL_DUT/Tx/DVB-S2 Tx/RRC Transmit Filter ==
  dataIn : Inport
  validIn : Inport  Port=2
  Discrete FIR Filter : dsphdlfiltering2/Discrete FIR Filter  NumeratorSource=Property  Numerator=config.RRCImpulseResponse  NumeratorPrototype=[]  FilterStructure=Direct form systolic  SerializationOption=Minimum number of cycles between valid input samples  NumCycles=2  NumberOfMultipliers=2  SimulateUsing=Code generation  roundingMode=Floor  overflowMode=off  CoefficientsDataTypeStr=Inherit: Same word length as input  OutputDataTypeStr=Inherit: Same word length as input  ResetInputPort=off  HDLGlobalReset=off  CoeffMultiplier=Multiplier  UseMultForPow2Coeff=on
  Repeat : dspsigops/Repeat  FactorSource=Dialog parameter  N=config.SamplesPerSymbol  Nmax=16  RateOptions=Allow multirate processing  ic=0  mode=Unused parameter value
  Upsample : dspsigops/Upsample  FactorSource=Dialog parameter  N=config.SamplesPerSymbol  Nmax=16  phase=0  RateOptions=Allow multirate processing  ic=0  mode=Unused parameter value
  dataOut : Outport
  validOut : Outport  Port=2
  wires:
  Discrete FIR Filter/2 -> validOut/1
  Discrete FIR Filter/1 -> dataOut/1
  dataIn/1 -> Upsample/1
  Upsample/1 -> Discrete FIR Filter/1
  validIn/1 -> Repeat/1
  Repeat/1 -> Discrete FIR Filter/2

== system dvbs2_stream/HDL_DUT/Tx/DVB-S2 Tx/Symbol Modulator ==
  dataIn : Inport
  startIn : Inport  Port=2
  endIn : Inport  Port=3
  validIn : Inport  Port=4
  FECFrame : Inport  Port=5
  codIdx : Inport  Port=6
  modIdx : Inport  Port=7
  MODCOD : Inport  Port=8
  DVB-S2 Symbol Modulator1 : whdlmod/DVB-S2 Symbol Modulator  ModulationSourceParams=Input port  ModulationScheme=QPSK  CodeRateAPSK=3/4  UnitAveragePower=off  SimulateUsing=Code generation  OutputDataType=Custom  WordLength=18
  Data Type Conversion : DataTypeConversion  OutDataTypeStr=fixdt(0,3,0)  SaturateOnIntegerOverflow=off  RndMeth=Floor
  Delay{,1..6,11,13} (9 alike) : Delay  DelayLength=1
  Delay{7..10,12,14} (6 alike) : Delay  DelayLength=3
  Delay{15..22} (8 alike) : Delay
  dataOut : Outport
  startOut : Outport  Port=2
  endOut : Outport  Port=3
  validOut : Outport  Port=4
  modIdxOut : Outport  Port=5
  codIdxOut : Outport  Port=6
  FECFrameOut : Outport  Port=7
  MODCODOut : Outport  Port=8
  wires:
  Data Type Conversion/1 -> DVB-S2 Symbol Modulator1/3
  DVB-S2 Symbol Modulator1/2 -> Delay16/1
  DVB-S2 Symbol Modulator1/1 -> Delay15/1
  Delay6/1 -> DVB-S2 Symbol Modulator1/5
  Delay1/1 -> DVB-S2 Symbol Modulator1/2
  Delay2/1 -> DVB-S2 Symbol Modulator1/1
  Delay22/1 -> FECFrameOut/1
  Delay21/1 -> MODCODOut/1
  Delay20/1 -> codIdxOut/1
  Delay19/1 -> modIdxOut/1
  Delay18/1 -> endOut/1
  Delay17/1 -> startOut/1
  Delay16/1 -> validOut/1
  Delay15/1 -> dataOut/1
  Delay14/1 -> Delay18/1
  Delay13/1 -> Delay14/1
  Delay12/1 -> Delay17/1
  Delay11/1 -> Delay12/1
  Delay10/1 -> Delay22/1
  Delay9/1 -> Delay21/1
  Delay8/1 -> Delay20/1
  Delay7/1 -> Delay19/1
  endIn/1 -> Delay13/1
  Delay5/1 -> Delay10/1
  FECFrame/1 -> Delay5/1
  Delay4/1 -> Delay9/1
  MODCOD/1 -> Delay4/1
  Delay3/1 -> Delay8/1, DVB-S2 Symbol Modulator1/4
  codIdx/1 -> Delay3/1
  startIn/1 -> Delay6/1, Delay11/1
  dataIn/1 -> Delay2/1
  validIn/1 -> Delay1/1
  Delay/1 -> Delay7/1, Data Type Conversion/1
  modIdx/1 -> Delay/1

== system dvbs2_stream/HDL_DUT/Tx/DVB-S2 Tx/BB Frame Generator/BB Header and Data CRC Generator ==
  dataIn : Inport
  startIn : Inport  Port=2
  endIn : Inport  Port=3
  validIn : Inport  Port=4
  frameEnd : Inport  Port=5
  frameStart : Inport  Port=6
  TSorGS : Inport  Port=7
  DFL : Inport  Port=8
  UPL : Inport  Port=9
  SYNC : Inport  Port=10
  MODCOD : Inport  Port=11
  FECFrame : Inport  Port=12
  BB Header Generator : Subsystem
  Data Field Generator : Subsystem
  Delay{,1..10} (11 alike) : Delay  DelayLength=1
  Logical Operator : Logic  Operator=OR  AllPortsSameDT=off  OutDataTypeStr=boolean
  Logical Operator1 : Logic  AllPortsSameDT=off  OutDataTypeStr=boolean
  Logical Operator2 : Logic  Operator=NOT  AllPortsSameDT=off  OutDataTypeStr=boolean
  MATLAB Function : MATLAB Function  TreatAsAtomicUnit=on
  No HDL : Subsystem
      settings: PortSchema="{\"entries\":[{\"content\":{\"sides\":[{\"content\":{\"connectorIds\":[\"In1\",\"In2\"]},\"type\":\"ConnectorPlacement.EquallySpacedRectSide\",\"uuid\":\"2b0d8642-5d0a-4928-807b-7bdaa72465a7\"},{\"content\":{\"connectorIds\":[\"In3\"],\"side\":\"RIGHT\"},\"type\":\"ConnectorPlacement.EquallySpacedRectSide\",\"uuid\":\"c3d25bc5-ada1-46aa-97a0-2934df92f89e\"},{\"content\":{\"side\":\"TOP\"},\"type\":\"ConnectorPlacement.EquallySpacedRectSide\",\"uuid\":\"4e9ad39f-657b-49f8-9193-07411e04c0d0\"},{\"content\":{\"side\":\"BOTTOM\"},\"type\":\"ConnectorPlacement.EquallySpacedRectSide\",\"uuid\":\"c9ac8116-ea00-4596-919b-501b9f95d4cb\"}]},\"type\":\"ConnectorPlacement.EquallySpacedConnector\",\"uuid\":\"3e308e49-dc99-4f24-8c75-1c979d051dde\"}],\"packageUris\":[\"http://schema.mathworks.com/mf0/Connector/R2020b\"],\"version\":\"1.0\"}"
  pktBits : Outport
  pktValid : Outport  Port=2
  DFLOut : Outport  Port=3
  bitsOut : Outport  Port=4
  startOut : Outport  Port=5
  endOut : Outport  Port=6
  validOut : Outport  Port=7
  MODCODOut : Outport  Port=8
  FECFrameOut : Outport  Port=9
  wires:
  Delay10/1 -> FECFrameOut/1
  BB Header Generator/7(FECFrameOut) -> Delay10/1
  FECFrame/1 -> BB Header Generator/7(FECFrame)
  Delay9/1 -> MODCODOut/1
  Delay8/1 -> endOut/1
  Delay7/1 -> validOut/1
  Delay6/1 -> startOut/1
  Delay5/1 -> bitsOut/1
  Delay4/1 -> MATLAB Function/4(DFL), DFLOut/1
  Delay3/1 -> MATLAB Function/3(endIn)
  Delay2/1 -> MATLAB Function/2(startIn)
  Delay1/1 -> Logical Operator/1, MATLAB Function/1(validIn)
  Delay/1 -> Logical Operator1/1
  MODCOD/1 -> BB Header Generator/6(MODCOD)
  BB Header Generator/6(MODCODOut) -> Delay9/1
  Logical Operator/1 -> pktValid/1
  Logical Operator1/1 -> pktBits/1
  Logical Operator2/1 -> Logical Operator1/2
  MATLAB Function/1(validAppend) -> No HDL/1(In2), Logical Operator2/1, Logical Operator/2
  Data Field Generator/3(frameStartOut) -> Delay2/1
  Data Field Generator/1(pktBits) -> Delay/1
  Data Field Generator/2(pktValid) -> Delay1/1
  BB Header Generator/1(DFLOut) -> Delay4/1
  BB Header Generator/5(endOut) -> Delay8/1
  frameEnd/1 -> Data Field Generator/5(frameEnd)
  SYNC/1 -> BB Header Generator/5(SYNC)
  frameStart/1 -> BB Header Generator/1(startIn), Data Field Generator/6(frameStart)
  BB Header Generator/3(startOut) -> Delay6/1
  dataIn/1 -> Data Field Generator/1(dataIn)
  startIn/1 -> Data Field Generator/2(startIn)
  Data Field Generator/4(frameEndOut) -> Delay3/1
  endIn/1 -> Data Field Generator/3(endIn)
  UPL/1 -> BB Header Generator/4(UPL), Data Field Generator/7(UPL)
  BB Header Generator/4(validOut) -> Delay7/1
  validIn/1 -> No HDL/3(vld), Data Field Generator/4(validIn)
  DFL/1 -> BB Header Generator/3(DFL)
  BB Header Generator/2(bitsOut) -> Delay5/1
  TSorGS/1 -> BB Header Generator/2(TSorGS)
  MATLAB Function/2(endAppend) -> No HDL/2(u)

== system dvbs2_stream/HDL_DUT/Tx/DVB-S2 Tx/BB Frame Generator/BB Scrambler ==
  bitsIn : Inport
  startIn : Inport  Port=2
  endIn : Inport  Port=3
  validIn : Inport  Port=4
  MODCOD : Inport  Port=5
  FECFrame : Inport  Port=6
  Data Type Conversion : DataTypeConversion  OutDataTypeStr=boolean  SaturateOnIntegerOverflow=off  RndMeth=Floor
  Delay{1..6} (6 alike) : Delay  DelayLength=1
  Logical Operator : Logic  Operator=XOR  AllPortsSameDT=off  OutDataTypeStr=boolean
  Subsystem : Subsystem
  bitsOut : Outport
  startOut : Outport  Port=2
  endOut : Outport  Port=3
  validOut : Outport  Port=4
  MODCODOut : Outport  Port=5
  FECFrameOut : Outport  Port=6
  wires:
  FECFrame/1 -> Delay6/1
  Delay6/1 -> FECFrameOut/1
  Delay4/1 -> MODCODOut/1
  Delay1/1 -> endOut/1
  Delay2/1 -> bitsOut/1
  Delay3/1 -> startOut/1
  Delay5/1 -> validOut/1
  MODCOD/1 -> Delay4/1
  Data Type Conversion/1 -> Logical Operator/1
  Logical Operator/1 -> Delay2/1
  startIn/1 -> Subsystem/1(In1), Delay3/1
  Subsystem/1(Out1) -> Data Type Conversion/1
  validIn/1 -> Subsystem/Enable, Delay5/1
  bitsIn/1 -> Logical Operator/2
  endIn/1 -> Delay1/1

== system dvbs2_stream/HDL_DUT/Tx/DVB-S2 Tx/BB Frame Generator/Data Store FIFO ==
  pktBits : Inport
  pktValid : Inport  Port=2
  DFLOut : Inport  Port=3
  bitsOut : Inport  Port=4
  startOut : Inport  Port=5
  endOut : Inport  Port=6
  validOut : Inport  Port=7
  MODCOD : Inport  Port=8
  FECFrame : Inport  Port=9
  Delay{,1..14} (15 alike) : Delay  DelayLength=1
  HDL Counter : hdlsllib/Sources/HDL Counter  CountType=Count limited  CountInit=0  CountStep=1  CountMax=2^7-1  CountFromType=Initial value  CountFrom=0  CountResetPort=off  CountLoadPort=off  CountEnbPort=on  CountDirPort=off  CountHitOutputPort=off  CountDataType=Unsigned  CountWordLen=7  CountFracLen=0  CountSampTime=1
  HDL Counter1 : hdlsllib/Sources/HDL Counter  CountType=Count limited  CountInit=0  CountStep=1  CountMax=2^7-1  CountFromType=Initial value  CountFrom=0  CountResetPort=off  CountLoadPort=off  CountEnbPort=on  CountDirPort=off  CountHitOutputPort=off  CountDataType=Unsigned  CountWordLen=7  CountFracLen=0  CountSampTime=1
  MATLAB Function : MATLAB Function  TreatAsAtomicUnit=on
  No HDL : Subsystem
  Simple Dual Port RAM : hdlsllib/HDL RAMs/Simple Dual Port RAM  ram_size=nextpow2(80)
  dataBits : Outport
  dataValid : Outport  Port=2
  dataEnd : Outport  Port=3
  headerBits : Outport  Port=4
  headerStart : Outport  Port=5
  headerValid : Outport  Port=6
  MODCODOut : Outport  Port=7
  FECFrameOut : Outport  Port=8
  wires:
  MATLAB Function/1(validOut) -> No HDL/1(rd), HDL Counter1/1, Delay/1
  Delay13/1 -> Delay14/1
  Delay14/1 -> FECFrameOut/1
  FECFrame/1 -> Delay13/1
  Delay12/1 -> MODCODOut/1
  Delay11/1 -> headerValid/1
  Delay10/1 -> headerStart/1
  Delay9/1 -> headerBits/1
  Delay8/1 -> dataEnd/1
  Delay7/1 -> dataValid/1
  Delay6/1 -> dataBits/1
  Delay5/1 -> Delay12/1
  MODCOD/1 -> Delay5/1
  Delay3/1 -> Delay10/1
  HDL Counter/1 -> Simple Dual Port RAM/2
  Delay4/1 -> Delay11/1
  Delay2/1 -> Delay9/1
  Delay1/1 -> Delay8/1
  Delay/1 -> Delay7/1
  MATLAB Function/2(endOut) -> Delay1/1
  HDL Counter1/1 -> Simple Dual Port RAM/4
  DFLOut/1 -> MATLAB Function/3(DFL)
  validOut/1 -> Delay4/1
  startOut/1 -> Delay3/1
  bitsOut/1 -> Delay2/1
  Simple Dual Port RAM/1 -> Delay6/1
  pktValid/1 -> No HDL/2(wr), HDL Counter/1, Simple Dual Port RAM/3, MATLAB Function/1(wr)
  pktBits/1 -> Simple Dual Port RAM/1
  endOut/1 -> MATLAB Function/2(startIn)
